simulink model "GFLIB_ControllerPIp_BAM_FLT"  (Simulink 7.3)
settings: Solver=ode45  StartTime=0.0  StopTime=10.0  RelTol=1e-3
undefined symbols (not defined in the file): fltIntegGain, fltPropGain
settings Model: Creator=RE004C  LastModifiedBy=RE004C
settings HardwareCC: ProdIntDivRoundTo=Zero  ProdEndianess=BigEndian  ProdHWDeviceType=Freescale->32-bit PowerPC

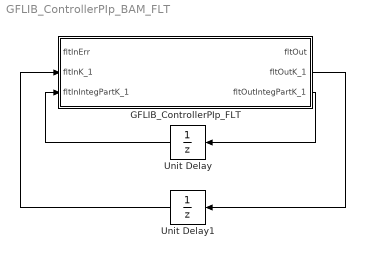
== system GFLIB_ControllerPIp_BAM_FLT ==
  GFLIB_ControllerPIp_FLT : Subsystem  mask(GFLIB_ControllerPIp_FLT){fltPropGain=fltPropGain, fltIntegGain=fltIntegGain}
      mask help: Bit accurate model of parallel form PI controller. All parameters as well as input and output are single precison floating point numbers with exception of u16LimitFlag, which is 16-bit unsigned integer.
      mask init:
      | pos = get_param(gcb, 'Position');width = pos(3) - pos(1); height = pos(4) - pos(2);tX=width/2;tY=height*0.9;
      mask Display:
      | color('black');
      | port_label('input',1,'fltInErr');
      | port_label('input',2,'fltInK_1');
      | port_label('input',3,'fltInIntegPartK_1');
      | port_label('output',1,'fltOut');
      | port_label('output',2,'fltOutK_1');
      | port_label('output',3,'fltOutIntegPartK_1');
      | color('black');
      | disp('GFLIB_ControllerPIp_FLT');
      | color('blue');
      | text(tX,tY, 'BAM', 'horizontalAlignment', 'center');
  Unit Delay : UnitDelay  SampleTime=-1
  Unit Delay1 : UnitDelay  SampleTime=-1
  wires:
  GFLIB_ControllerPIp_FLT/3(fltOutIntegPartK_1) -> Unit Delay/1
  Unit Delay/1 -> GFLIB_ControllerPIp_FLT/3(fltInIntegPartK_1)
  GFLIB_ControllerPIp_FLT/2(fltOutK_1) -> Unit Delay1/1
  Unit Delay1/1 -> GFLIB_ControllerPIp_FLT/2(fltInK_1)

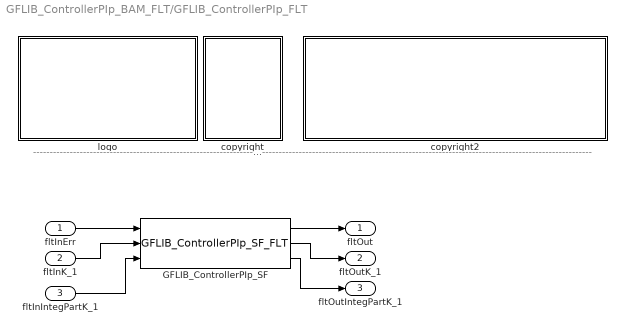
== system GFLIB_ControllerPIp_BAM_FLT/GFLIB_ControllerPIp_FLT ==
  note: ---------------------------------------------------------------------------------------------------------------------------------------------------------------------------------------------------
  fltInErr : Inport  OutDataType=fixdt(1, 16)  OutScaling=2^0
  fltInK_1 : Inport  Port=2  OutDataType=fixdt(1, 16)  OutScaling=2^0
  fltInIntegPartK_1 : Inport  Port=3  OutDataType=fixdt(1, 16)  OutScaling=2^0
  GFLIB_ControllerPIp_SF : S-Function  FunctionName=GFLIB_ControllerPIp_SF_FLT  Parameters=fltPropGain,fltIntegGain  EnableBusSupport=off
  copyright : Subsystem
      mask Display: text(10,90,'FILE:');text(10,75,'DESRIPTION:')text(10,60,'COPYRIGHT:')text(10,45,'VERSION:')text(10,30,'DATE:')
  copyright2 : Subsystem
      mask Display: text(10,90,'GFLIB_ControllerPIp_BAM_FLT.mdl');text(10,75,'Parallel form of a standard PI controller without implemented anti-windup.');text(10,60,'Freescale')text(10,45,'0.1');text(10,30,'20-Jan-2012');
  logo : Subsystem
      mask Display: image(imread('logo.jpg'))
  fltOut : Outport  OutDataType=fixdt(1, 16)  OutScaling=2^0
  fltOutK_1 : Outport  Port=2  OutDataType=fixdt(1, 16)  OutScaling=2^0
  fltOutIntegPartK_1 : Outport  Port=3  OutDataType=fixdt(1, 16)  OutScaling=2^0
  wires:
  fltInErr/1 -> GFLIB_ControllerPIp_SF/1
  GFLIB_ControllerPIp_SF/1 -> fltOut/1
  GFLIB_ControllerPIp_SF/2 -> fltOutK_1/1
  GFLIB_ControllerPIp_SF/3 -> fltOutIntegPartK_1/1
  fltInK_1/1 -> GFLIB_ControllerPIp_SF/2
  fltInIntegPartK_1/1 -> GFLIB_ControllerPIp_SF/3

== system GFLIB_ControllerPIp_BAM_FLT/GFLIB_ControllerPIp_FLT/copyright ==

== system GFLIB_ControllerPIp_BAM_FLT/GFLIB_ControllerPIp_FLT/copyright2 ==

== system GFLIB_ControllerPIp_BAM_FLT/GFLIB_ControllerPIp_FLT/logo ==
